simulink model "AutoHeadlightControl"  (R2025b)
settings: Solver=FixedStepDiscrete  StartTime=0.0  StopTime=40  FixedStep=0.1  RelTol=1e-3
libraries: hdlsllib x3
settings Model: Creator=Palash  LastModifiedBy=Palash
settings DataIOCC: SaveFormat=StructureWithTime

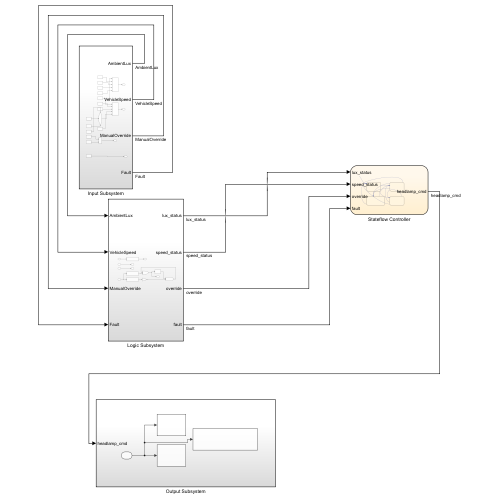
[thumbnail: Simulink's stored preview of the top-level diagram]
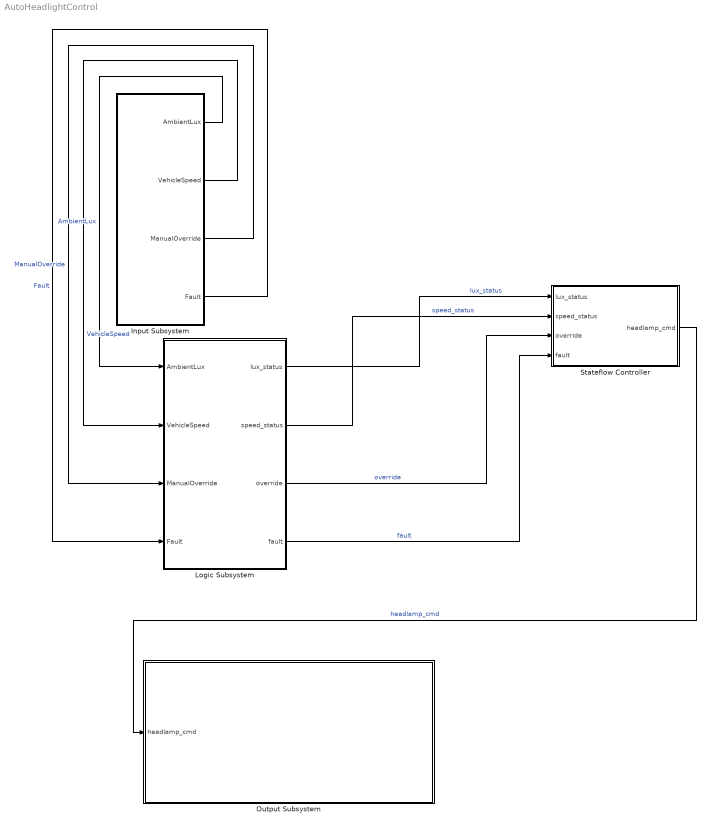
== system AutoHeadlightControl ==
  Input Subsystem : Subsystem
  Logic Subsystem : Subsystem
  Output Subsystem : Subsystem
  Stateflow Controller : Stateflow chart  TreatAsAtomicUnit=on  SystemSampleTime=0.1
  wires:
  Input Subsystem/1(AmbientLux) -> Logic Subsystem/1(AmbientLux)  "AmbientLux"
  Input Subsystem/2(VehicleSpeed) -> Logic Subsystem/2(VehicleSpeed)  "VehicleSpeed"
  Input Subsystem/3(ManualOverride) -> Logic Subsystem/3(ManualOverride)  "ManualOverride"
  Input Subsystem/4(Fault) -> Logic Subsystem/4(Fault)  "Fault"
  Logic Subsystem/1(lux_status) -> Stateflow Controller/1(lux_status)  "lux_status"
  Logic Subsystem/2(speed_status) -> Stateflow Controller/2(speed_status)  "speed_status"
  Logic Subsystem/3(override) -> Stateflow Controller/3(override)  "override"
  Logic Subsystem/4(fault) -> Stateflow Controller/4(fault)  "fault"
  Stateflow Controller/1(headlamp_cmd) -> Output Subsystem/1(headlamp_cmd)  "headlamp_cmd"

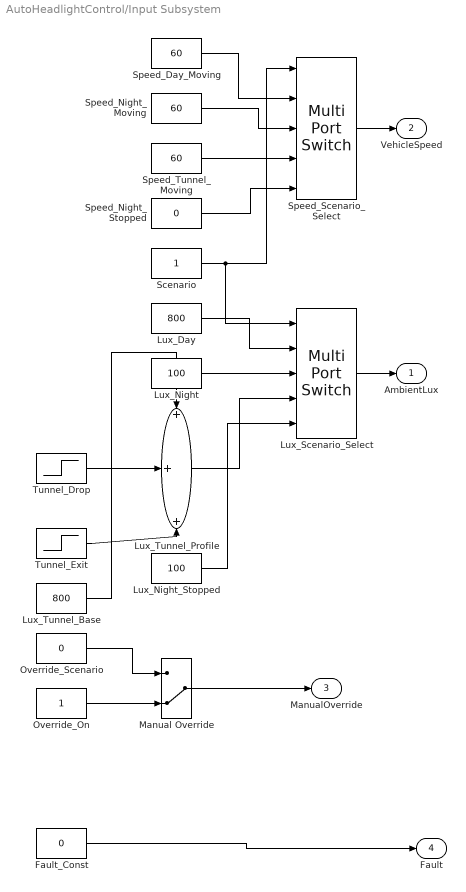
== system AutoHeadlightControl/Input Subsystem ==
  Fault_Const : Constant  Value=0  OutDataTypeStr=boolean
  Lux_Day : Constant  Value=800
  Lux_Night : Constant  Value=100
  Lux_Night_Stopped : Constant  Value=100
  Lux_Scenario_Select : MultiPortSwitch  Inputs=4  SaturateOnIntegerOverflow=off  InputSameDT=off
  Lux_Tunnel_Base : Constant  Value=800
  Lux_Tunnel_Profile : Sum  Inputs=+++
  Manual Override : ManualSwitch  CurrentSetting=0
  Override_On : Constant  OutDataTypeStr=boolean
  Override_Scenario : Constant  Value=0  OutDataTypeStr=boolean
  Scenario : Constant
  Speed_Day_Moving : Constant  Value=60
  Speed_Night_Moving : Constant  Value=60
  Speed_Night_Stopped : Constant  Value=0
  Speed_Scenario_Select : MultiPortSwitch  Inputs=4  SaturateOnIntegerOverflow=off  InputSameDT=off
  Speed_Tunnel_Moving : Constant  Value=60
  Tunnel_Drop : Step  Time=10  After=-700  SampleTime=0.1
  Tunnel_Exit : Step  Time=20  After=700  SampleTime=0.1
  AmbientLux : Outport
  VehicleSpeed : Outport  Port=2
  ManualOverride : Outport  Port=3
  Fault : Outport  Port=4
  wires:
  Lux_Tunnel_Base/1 -> Lux_Tunnel_Profile/1
  Tunnel_Drop/1 -> Lux_Tunnel_Profile/2
  Tunnel_Exit/1 -> Lux_Tunnel_Profile/3
  Scenario/1 -> Speed_Scenario_Select/1, Lux_Scenario_Select/1
  Lux_Day/1 -> Lux_Scenario_Select/2
  Lux_Night/1 -> Lux_Scenario_Select/3
  Lux_Tunnel_Profile/1 -> Lux_Scenario_Select/4
  Lux_Night_Stopped/1 -> Lux_Scenario_Select/5
  Speed_Day_Moving/1 -> Speed_Scenario_Select/2
  Speed_Night_Moving/1 -> Speed_Scenario_Select/3
  Speed_Tunnel_Moving/1 -> Speed_Scenario_Select/4
  Speed_Night_Stopped/1 -> Speed_Scenario_Select/5
  Override_Scenario/1 -> Manual Override/1
  Override_On/1 -> Manual Override/2
  Lux_Scenario_Select/1 -> AmbientLux/1
  Speed_Scenario_Select/1 -> VehicleSpeed/1
  Manual Override/1 -> ManualOverride/1
  Fault_Const/1 -> Fault/1

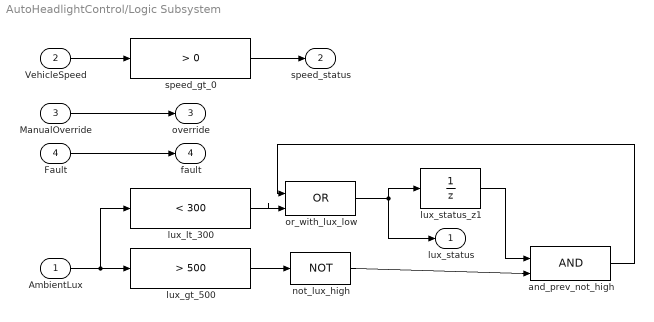
== system AutoHeadlightControl/Logic Subsystem ==
  AmbientLux : Inport
  VehicleSpeed : Inport  Port=2
  ManualOverride : Inport  Port=3
  Fault : Inport  Port=4
  and_prev_not_high : Logic  IconShape=distinctive  AllPortsSameDT=off  OutDataTypeStr=boolean
  lux_gt_500 : hdlsllib/Logic and Bit Operations/Compare To Constant  relop=>  const=500  OutDataTypeStr=boolean
  lux_lt_300 : hdlsllib/Logic and Bit Operations/Compare To Constant  relop=<  const=300  OutDataTypeStr=boolean
  lux_status_z1 : UnitDelay  SampleTime=-1  HasFrameUpgradeWarning=on
  not_lux_high : Logic  Operator=NOT  IconShape=distinctive  AllPortsSameDT=off  OutDataTypeStr=boolean
  or_with_lux_low : Logic  Operator=OR  IconShape=distinctive  AllPortsSameDT=off  OutDataTypeStr=boolean
  speed_gt_0 : hdlsllib/Logic and Bit Operations/Compare To Constant  relop=>  const=0  OutDataTypeStr=boolean
  lux_status : Outport
  speed_status : Outport  Port=2
  override : Outport  Port=3
  fault : Outport  Port=4
  wires:
  AmbientLux/1 -> lux_gt_500/1, lux_lt_300/1
  VehicleSpeed/1 -> speed_gt_0/1
  lux_gt_500/1 -> not_lux_high/1
  lux_status_z1/1 -> and_prev_not_high/1
  not_lux_high/1 -> and_prev_not_high/2
  and_prev_not_high/1 -> or_with_lux_low/1
  lux_lt_300/1 -> or_with_lux_low/2
  or_with_lux_low/1 -> lux_status_z1/1, lux_status/1
  speed_gt_0/1 -> speed_status/1
  ManualOverride/1 -> override/1
  Fault/1 -> fault/1

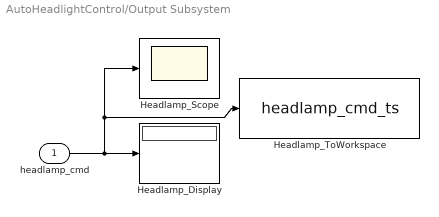
== system AutoHeadlightControl/Output Subsystem ==
  headlamp_cmd : Inport
  Headlamp_Display : Display
  Headlamp_Scope : Scope
      settings: ActiveDisplayYMinimum=-1  ActiveDisplayYMaximum=1
  Headlamp_ToWorkspace : ToWorkspace  VariableName=headlamp_cmd_ts  SaveFormat=Timeseries
  wires:
  headlamp_cmd/1 -> Headlamp_ToWorkspace/1, Headlamp_Scope/1, Headlamp_Display/1

== stateflow chart AutoHeadlightControl/Stateflow Controller ==
  settings: updateMethod=DISCRETE  sampleTime=0.1
  state OFF
    entry: headlamp_cmd = fault;
    during: headlamp_cmd = fault;
  state ON
    entry: headlamp_cmd = true;
    during: headlamp_cmd = true;
  state MANUAL
    entry: headlamp_cmd = true;
    during: headlamp_cmd = true;
  state HOLD
    entry: headlamp_cmd = true;
    during: headlamp_cmd = true;
  (default) -> OFF
  ON -> OFF [order 2] : [~override && (~lux_status || ~speed_status)]
  MANUAL -> OFF [order 2] : [~override && (~lux_status || ~speed_status)]
  HOLD -> OFF [order 3] : [~override && ~lux_status]
  ON -> MANUAL [order 1] : [override]
  MANUAL -> ON [order 1] : [~override && lux_status && speed_status]
  OFF -> ON [order 2] : [~override && lux_status && speed_status]
  HOLD -> ON [order 2] : [~override && lux_status && speed_status]
  HOLD -> MANUAL [order 1] : [override]
  ON -> HOLD [order 3] : [~override && lux_status && ~speed_status]
  OFF -> MANUAL [order 1] : [override]
  OFF -> HOLD [order 3] : [~override && lux_status && ~speed_status]
  data: lux_status input boolean; speed_status input boolean; override input boolean; fault input boolean; headlamp_cmd output boolean
